simulink model "unicycle_model"  (R2024a)
settings: Solver=ode4  StartTime=0.0  StopTime=4000  FixedStep=0.001  RelTol=1e-10  AbsTol=1e-10
values from neighbouring files (symbols this model uses):
  a1 = 5e-6    (= 5e-06)    [quadcopter_param.m]    (also in satellite_param.m = ab1 / I(1,1); unicycle_param.m = 4e-05)
  a2 = 7.5e-6    (= 7.5e-06)    [quadcopter_param.m]    (also in satellite_param.m = ab2 / I(2,2); unicycle_param.m = 0.0052)
  c1 = 0.154    [quadcopter_param.m]    (also in satellite_param.m = cb1 / I(1,1); unicycle_param.m = 0.4)
  c2 = 0.237    [quadcopter_param.m]    (also in satellite_param.m = cb2 / I(2,2); unicycle_param.m = 2.4)
  delay = 0.01    [quadcopter_param.m]    (also in satellite_param.m = 0.003; unicycle_param.m)
  k = 3.95    [quadcopter_param.m]    (also in satellite_param.m = 2.4; unicycle_param.m = 12.5)
  omega = 25    [quadcopter_param.m]    (also in satellite_param.m = 36; unicycle_param.m = 50)
  variance = 1e-6    (= 1e-06)    [quadcopter_param.m]    (also in satellite_param.m = 1e-09; unicycle_param.m)
settings Model: Creator=rohan  LastModifiedBy=rohan

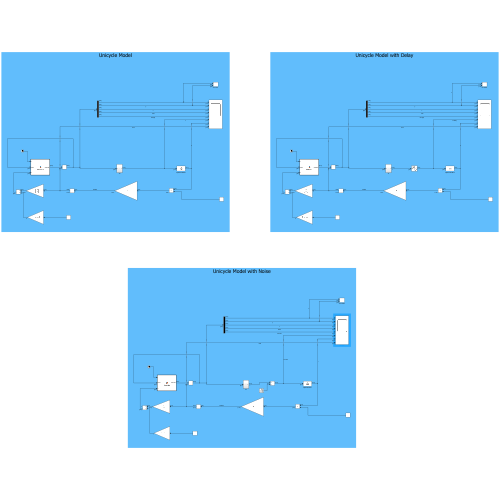
[thumbnail: Simulink's stored preview of the top-level diagram]
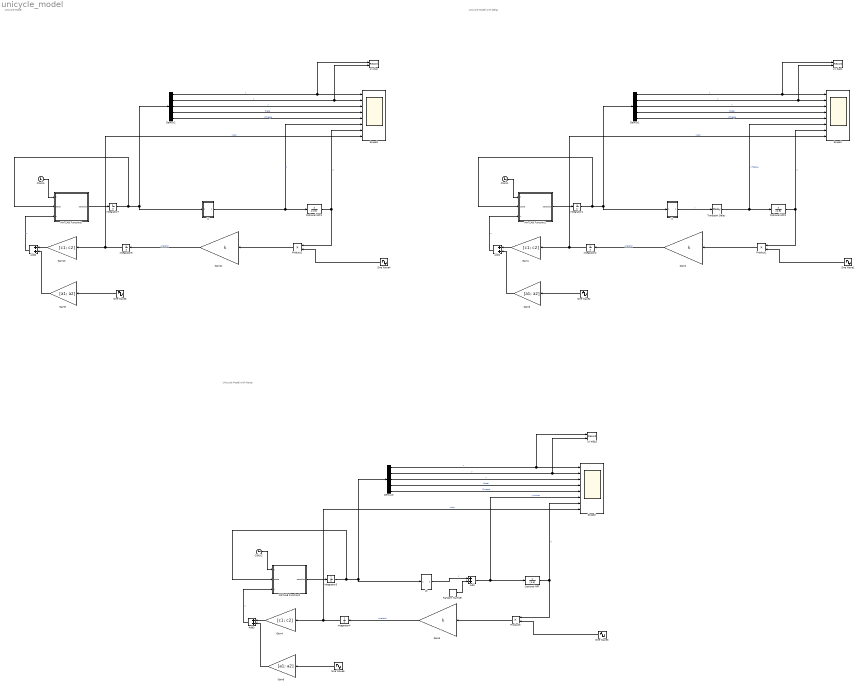
== system unicycle_model ==
  note: Unicycle Model
  note: Unicycle Model with Delay
  note: Unicycle Model with Noise
  Add{,1..3} (4 alike) : Sum
  Clock1 : Clock
  Clock2 : Clock
  Clock3 : Clock
  Demux1 : Demux  Outputs=5
  Demux2 : Demux  Outputs=5
  Demux3 : Demux  Outputs=5
  Gain1 : Gain  Gain=[c1; c2]
  Gain10 : Gain  Gain=[c1; c2]
  Gain11 : Gain  Gain=k
  Gain2 : Gain  Gain=k
  Gain3 : Gain  Gain=[a1; a2]
  Gain4 : Gain  Gain=[c1; c2]
  Gain5 : Gain  Gain=k
  Gain6 : Gain  Gain=[a1; a2]
  Gain9 : Gain  Gain=[a1; a2]
  Integrator1 : Integrator  InitialCondition=[2;2;0;0;1.5]
  Integrator2 : Integrator
  Integrator3 : Integrator  InitialCondition=[2;2;0;0;1.5]
  Integrator4 : Integrator
  Integrator7 : Integrator  InitialCondition=[2;2;0;0;1.5]
  Integrator9 : Integrator
  J1 : Subsystem
  J2 : Subsystem
  J3 : Subsystem
  MATLAB Function1 : MATLAB Function  TreatAsAtomicUnit=on
  MATLAB Function2 : MATLAB Function  TreatAsAtomicUnit=on
  MATLAB Function5 : MATLAB Function  TreatAsAtomicUnit=on
  Optional HPF : TransferFcn  Numerator=[1 0]  Denominator=[1 e]
  Optional HPF1 : TransferFcn  Numerator=[1 0]  Denominator=[1 e]
  Optional HPF2 : TransferFcn  Numerator=[1 0]  Denominator=[1 e]
  Product1 : Product
  Product2 : Product
  Product3 : Product
  Random Number : RandomNumber  Variance=variance  Seed=1  SampleTime=0.001
  Scope1 : Scope  NumInputPorts=8
  Scope2 : Scope  NumInputPorts=8
  Scope3 : Scope  NumInputPorts=8
  Sine Wave{1..6} (6 alike) : Sin  Amplitude=omega  Frequency=omega  Phase=pi/2  SampleTime=0
  Transport Delay : TransportDelay  DelayTime=delay  InitialOutput=(2-1)^2 + (2-1)^2
  XY Plot : Record  FileSettingsInternal="{\"entries\":[{\"content\":{\"excelSettings\":{\"content\":{},\"type\":\"Streamout.ExcelSettings\"}},\"type\":\"Streamout.FileSettingStorage\",\"uuid\":\"\"}],\"packageUris\":[\"http:\\/\\/schema.mathworks.com\\/mf0\\/streamout_blocks\\/R2020a\"],\"version\":\"1.0\"}"  Layout=[1 1]  SignalsInternal="{\"entries\":[{\"content\":{\"signals\":[{\"content\":{\"blockPath\":[],\"dimensions\":[1,1],\"domain\":\"\",\"lineColor\":\"#64d413\",\"lineWidth\":2,\"port\":1,\"sid\":[\"\"],\"signalID\":1,\"signalName\":\"x\"},\"type\":\"RecordBlkView.Signal\",\"uuid\":\"\"},{\"content\":{\"blockPath\":[],\"dimensions\":[1,1],\"domain\":\"\",\"lineColor\":\"#ff13a6\",\"lineWidth\":2,\"port\":2,\"sid\":[\"\"],\"signalID\":2,\"signalName\":\"y\"},\"type\":\"RecordBlkView.Signal\",\"uuid\":\"\"}]},\"type\":\"RecordBlkView.InputSignals\",\"uuid\":\"\"}],\"packageUris\":[\"http:\\/\\/schema.mathworks.com\\/mf0\\/streamout_blocks\\/R2020a\"],\"version\":\"1.0\"}"  VisualizationBindings="{\"xyplotplugin\":{\"info\":[{\"series\":[],\"subplotID\":1}]}}"  CompatibilityTag=XY
  XY Plot1 : Record  FileSettingsInternal="{\"entries\":[{\"content\":{\"excelSettings\":{\"content\":{},\"type\":\"Streamout.ExcelSettings\"}},\"type\":\"Streamout.FileSettingStorage\",\"uuid\":\"\"}],\"packageUris\":[\"http:\\/\\/schema.mathworks.com\\/mf0\\/streamout_blocks\\/R2020a\"],\"version\":\"1.0\"}"  Layout=[1 1]  SignalsInternal="{\"entries\":[{\"content\":{\"signals\":[{\"content\":{\"blockPath\":[],\"dimensions\":[1,1],\"domain\":\"\",\"lineColor\":\"#ff6929\",\"lineWidth\":2,\"port\":1,\"sid\":[\"\"],\"signalID\":1,\"signalName\":\"x\"},\"type\":\"RecordBlkView.Signal\",\"uuid\":\"\"},{\"content\":{\"blockPath\":[],\"dimensions\":[1,1],\"domain\":\"\",\"lineColor\":\"#b746ff\",\"lineWidth\":2,\"port\":2,\"sid\":[\"\"],\"signalID\":2,\"signalName\":\"y\"},\"type\":\"RecordBlkView.Signal\",\"uuid\":\"\"}]},\"type\":\"RecordBlkView.InputSignals\",\"uuid\":\"\"}],\"packageUris\":[\"http:\\/\\/schema.mathworks.com\\/mf0\\/streamout_blocks\\/R2020a\"],\"version\":\"1.0\"}"  VisualizationBindings="{\"xyplotplugin\":{\"info\":[{\"series\":[],\"subplotID\":1}]}}"  CompatibilityTag=XY
  XY Plot2 : Record  FileSettingsInternal="{\"entries\":[{\"content\":{\"excelSettings\":{\"content\":{},\"type\":\"Streamout.ExcelSettings\"}},\"type\":\"Streamout.FileSettingStorage\",\"uuid\":\"\"}],\"packageUris\":[\"http:\\/\\/schema.mathworks.com\\/mf0\\/streamout_blocks\\/R2020a\"],\"version\":\"1.0\"}"  Layout=[1 1]  SignalsInternal="{\"entries\":[{\"content\":{\"signals\":[{\"content\":{\"blockPath\":[],\"dimensions\":[1,1],\"domain\":\"\",\"lineColor\":\"#a2142f\",\"lineWidth\":2,\"port\":1,\"sid\":[\"\"],\"signalID\":1,\"signalName\":\"x\"},\"type\":\"RecordBlkView.Signal\",\"uuid\":\"\"},{\"content\":{\"blockPath\":[],\"dimensions\":[1,1],\"domain\":\"\",\"lineColor\":\"#139fff\",\"lineWidth\":2,\"port\":2,\"sid\":[\"\"],\"signalID\":2,\"signalName\":\"y\"},\"type\":\"RecordBlkView.Signal\",\"uuid\":\"\"}]},\"type\":\"RecordBlkView.InputSignals\",\"uuid\":\"\"}],\"packageUris\":[\"http:\\/\\/schema.mathworks.com\\/mf0\\/streamout_blocks\\/R2020a\"],\"version\":\"1.0\"}"  VisualizationBindings="{\"xyplotplugin\":{\"info\":[{\"series\":[],\"subplotID\":1}]}}"  CompatibilityTag=XY
  wires:
  MATLAB Function5/1(statedot) -> Integrator7/1
  Integrator7/1 -> MATLAB Function5/2(state), J2/1(In1), Demux2/1
  J2/1(Out1) -> Optional HPF1/1, Scope3/6  "J"
  Sine Wave4/1 -> Product2/2
  Product2/1 -> Gain11/1
  Integrator9/1 -> Scope3/8, Gain10/1  "uhat"
  Gain9/1 -> Add2/2
  Add2/1 -> MATLAB Function5/3(u)  "u"
  Clock3/1 -> MATLAB Function5/1(t)
  Demux2/1 -> XY Plot/1, Scope3/1  "x"
  Demux2/2 -> XY Plot/2, Scope3/2  "y"
  Demux2/3 -> Scope3/3  "v"
  Demux2/4 -> Scope3/4  "theta"
  Demux2/5 -> Scope3/5  "Omega"
  Gain10/1 -> Add2/1
  Optional HPF1/1 -> Product2/1, Scope3/7  "h"
  Gain11/1 -> Integrator9/1  "uhatdot"
  Sine Wave5/1 -> Gain9/1
  Demux1/1 -> XY Plot1/1, Scope1/1  "x"
  Integrator1/1 -> MATLAB Function1/2(state), J1/1(In1), Demux1/1
  J1/1(Out1) -> Transport Delay/1  "J"
  Demux1/4 -> Scope1/4  "theta"
  Optional HPF2/1 -> Product1/1, Scope1/7  "h"
  MATLAB Function1/1(statedot) -> Integrator1/1
  Gain1/1 -> Add1/1
  Sine Wave1/1 -> Product1/2
  Integrator2/1 -> Scope1/8, Gain1/1  "uhat"
  Gain3/1 -> Add1/2
  Product1/1 -> Gain2/1
  Demux1/5 -> Scope1/5  "Omega"
  Demux1/3 -> Scope1/3  "v"
  Add1/1 -> MATLAB Function1/3(u)  "u"
  Clock1/1 -> MATLAB Function1/1(t)
  Gain2/1 -> Integrator2/1  "uhatdot"
  Sine Wave2/1 -> Gain3/1
  Demux1/2 -> XY Plot1/2, Scope1/2  "y"
  Demux3/2 -> Scope2/2, XY Plot2/2  "y"
  Sine Wave6/1 -> Gain6/1
  Gain5/1 -> Integrator4/1  "uhatdot"
  Clock2/1 -> MATLAB Function2/1(t)
  Add3/1 -> MATLAB Function2/3(u)  "u"
  Demux3/3 -> Scope2/3  "v"
  Demux3/5 -> Scope2/5  "Omega"
  Product3/1 -> Gain5/1
  Gain6/1 -> Add3/2
  Integrator4/1 -> Gain4/1, Scope2/8  "uhat"
  Sine Wave3/1 -> Product3/2
  Gain4/1 -> Add3/1
  MATLAB Function2/1(statedot) -> Integrator3/1
  Optional HPF/1 -> Product3/1, Scope2/7  "h"
  Demux3/4 -> Scope2/4  "theta"
  Integrator3/1 -> Demux3/1, J3/1(In1), MATLAB Function2/2(state)
  Demux3/1 -> Scope2/1, XY Plot2/1  "x"
  Transport Delay/1 -> Optional HPF2/1, Scope1/6  "J+delay"
  J3/1(Out1) -> Add/1  "J"
  Random Number/1 -> Add/2
  Add/1 -> Scope2/6, Optional HPF/1  "J+noise"

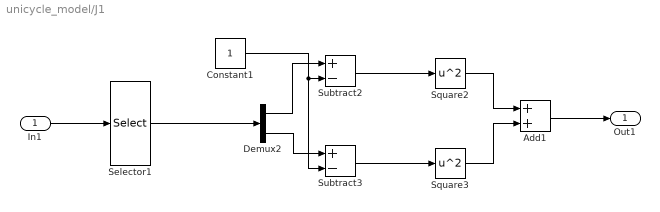
== system unicycle_model/J1 ==
  In1 : Inport
  Add1 : Sum
  Constant1 : Constant
  Demux2 : Demux  Outputs=2
  Selector1 : Selector  InputPortWidth=5  IndexOptions=Index vector (dialog)  Indices=[1 2]  OutputSizes=1
  Square2 : Math  Operator=square
  Square3 : Math  Operator=square
  Subtract2 : Sum  Inputs=+-
  Subtract3 : Sum  Inputs=+-
  Out1 : Outport
  wires:
  Demux2/1 -> Subtract2/1
  Selector1/1 -> Demux2/1
  Constant1/1 -> Subtract3/2, Subtract2/2
  Square2/1 -> Add1/1
  Square3/1 -> Add1/2
  Demux2/2 -> Subtract3/1
  Subtract3/1 -> Square3/1
  Subtract2/1 -> Square2/1
  Add1/1 -> Out1/1
  In1/1 -> Selector1/1

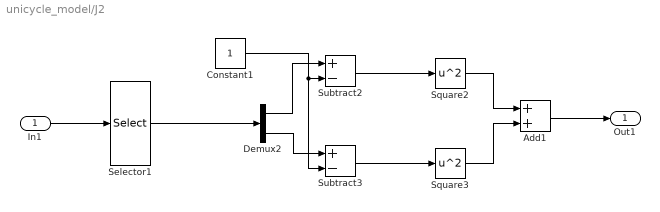
== system unicycle_model/J2 ==
  In1 : Inport
  Add1 : Sum
  Constant1 : Constant
  Demux2 : Demux  Outputs=2
  Selector1 : Selector  InputPortWidth=5  IndexOptions=Index vector (dialog)  Indices=[1 2]  OutputSizes=1
  Square2 : Math  Operator=square
  Square3 : Math  Operator=square
  Subtract2 : Sum  Inputs=+-
  Subtract3 : Sum  Inputs=+-
  Out1 : Outport
  wires:
  Demux2/1 -> Subtract2/1
  Selector1/1 -> Demux2/1
  Constant1/1 -> Subtract3/2, Subtract2/2
  Square2/1 -> Add1/1
  Square3/1 -> Add1/2
  Demux2/2 -> Subtract3/1
  Subtract3/1 -> Square3/1
  Subtract2/1 -> Square2/1
  Add1/1 -> Out1/1
  In1/1 -> Selector1/1

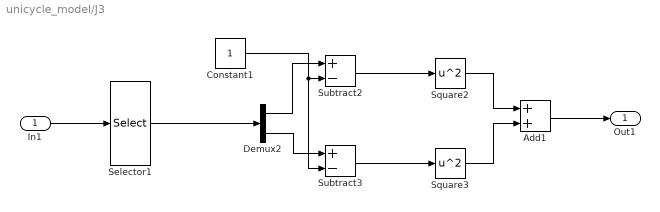
== system unicycle_model/J3 ==
  In1 : Inport
  Add1 : Sum
  Constant1 : Constant
  Demux2 : Demux  Outputs=2
  Selector1 : Selector  InputPortWidth=5  IndexOptions=Index vector (dialog)  Indices=[1 2]  OutputSizes=1
  Square2 : Math  Operator=square
  Square3 : Math  Operator=square
  Subtract2 : Sum  Inputs=+-
  Subtract3 : Sum  Inputs=+-
  Out1 : Outport
  wires:
  In1/1 -> Selector1/1
  Add1/1 -> Out1/1
  Subtract2/1 -> Square2/1
  Subtract3/1 -> Square3/1
  Demux2/2 -> Subtract3/1
  Square3/1 -> Add1/2
  Square2/1 -> Add1/1
  Constant1/1 -> Subtract2/2, Subtract3/2
  Selector1/1 -> Demux2/1
  Demux2/1 -> Subtract2/1

== matlab function unicycle_model/MATLAB Function2 ==
  data: t input; statedot output; state input; u input
function statedot = dynamics(t,state,u)
xpos = state(1);
ypos = state(2);
v = state(3);
theta = state(4);
Omega = state(5);

d1 = 0.2;
d2 = 0.1;

xdot = v * cos(theta);
ydot = v * sin(theta);
vdot = u(1) - d1*v;
thetadot = Omega;
Omegadot = u(2) - d2*Omega;

statedot = [xdot; ydot; vdot; thetadot; Omegadot];

== matlab function unicycle_model/MATLAB Function5 ==
  data: t input; statedot output; state input; u input
function statedot = dynamics(t,state,u)
xpos = state(1);
ypos = state(2);
v = state(3);
theta = state(4);
Omega = state(5);

d1 = 0.2;
d2 = 0.1;

xdot = v * cos(theta);
ydot = v * sin(theta);
vdot = u(1) - d1*v;
thetadot = Omega;
Omegadot = u(2) - d2*Omega;

statedot = [xdot; ydot; vdot; thetadot; Omegadot];

== matlab function unicycle_model/MATLAB Function1 ==
  data: t input; statedot output; state input; u input
function statedot = dynamics(t,state,u)
xpos = state(1);
ypos = state(2);
v = state(3);
theta = state(4);
Omega = state(5);

d1 = 0.2;
d2 = 0.1;

xdot = v * cos(theta);
ydot = v * sin(theta);
vdot = u(1) - d1*v;
thetadot = Omega;
Omegadot = u(2) - d2*Omega;

statedot = [xdot; ydot; vdot; thetadot; Omegadot];
